simulink model "unlinear1130"  (R2021a)
settings: Solver=ode45  StartTime=0.0  StopTime=20  FixedStep=0  RelTol=1e-3  EnableMultiTasking=on
libraries: pid_lib x19, simulink x19
settings Model: NumberOfSteps=2  Creator=secn18  LastModifiedBy=HanDong
settings SolverCC: AlgebraicLoopSolver=TrustRegion
settings DataIOCC: LimitDataPoints=on  SaveFormat=Array  ReturnWorkspaceOutputs=off
settings OptimizationCC: LifeSpan=inf
settings DebuggingCC: SolverPrmCheckMsg=warning  SFUnexpectedBacktrackingDiag=warning  SFNoUnconditionalDefaultTransitionDiag=warning  SFExecutionAtInitializationDiag=none  SFMachineParentedDataDiag=warning  ArithmeticOperatorsInVariantConditions=warning
settings HardwareCC: ProdBitPerPointer=32  ProdBitPerSizeT=32  ProdBitPerPtrDiffT=32  ProdLargestAtomicFloat=None  ProdIntDivRoundTo=Undefined  ProdEndianess=Unspecified  ProdWordSize=32  ProdHWDeviceType=32-bit Generic
settings ModelReferenceCC: PropagateSignalLabelsOutOfModel=off
settings SFSimCC: SimUseLocalCustomCode=off  CustomCodeUndefinedFunction=UseInterfaceOnly
settings RTWCC: RTWUseLocalCustomCode=off
settings CodeAppCC: StateflowObjectComments=on
settings GRTTargetCC: TargetLangStandard=C89/C90 (ANSI)
settings ConfigComp: CovMetricSettings=dw  CovSaveCumulativeToWorkspaceVar=on  CovSaveSingleToWorkspaceVar=on  CovExternalEMLEnable=off  CovSFcnEnable=off

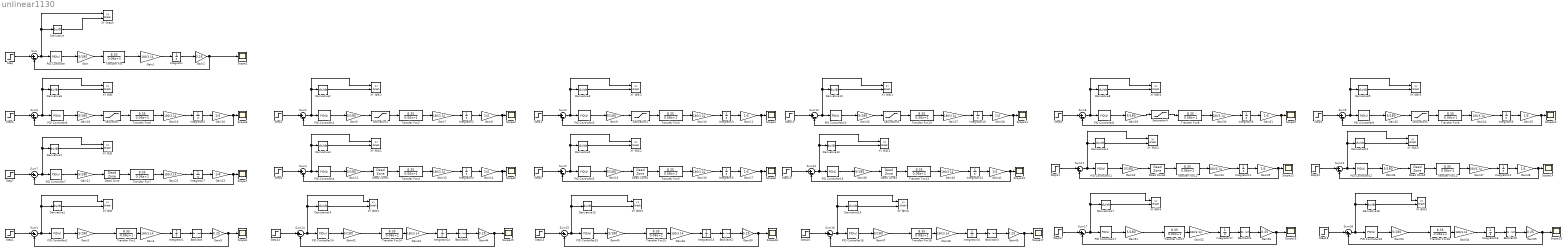
== system unlinear1130 ==
  Backlash : Backlash  BacklashWidth=0.2
  Backlash1 : Backlash  BacklashWidth=0.3
  Backlash2 : Backlash  BacklashWidth=0.4
  Backlash3 : Backlash  BacklashWidth=0.5
  Backlash4 : Backlash  BacklashWidth=1.2
  Backlash5 : Backlash  BacklashWidth=5
  Dead Zone : DeadZone  LowerValue=-0.2  UpperValue=0.2  SaturateOnIntegerOverflow=on
  Dead Zone1 : DeadZone  LowerValue=-0.3  UpperValue=0.3  SaturateOnIntegerOverflow=on
  Dead Zone2 : DeadZone  LowerValue=-0.4  UpperValue=0.4  SaturateOnIntegerOverflow=on
  Dead Zone3 : DeadZone  LowerValue=-1  UpperValue=1  SaturateOnIntegerOverflow=on
  Dead Zone4 : DeadZone  LowerValue=-5  UpperValue=5  SaturateOnIntegerOverflow=on
  Dead Zone5 : DeadZone  LowerValue=-10  UpperValue=10  SaturateOnIntegerOverflow=on
  Derivative{,1..18} (19 alike) : Derivative
  Gain{,3,6,9,12,15,18,21,26,29,32..33,36,39,42,45,47,51,53} (19 alike) : Gain  Gain=5/180
  Gain{1,4,7,10,13,16,19,22,24,27,30,34,37,40,43,46,48,52,54} (19 alike) : Gain  Gain=180/3.14
  Gain{8,11,14,17,20,23,25,28,31,35,38,41} (12 alike) : Gain  Gain=1/4
  Gain{2,5,44,49..50,55..56} (7 alike) : Gain  Gain=0.25
  Integrator{,1..18} (19 alike) : Integrator
  PID Controller : pid_lib/PID Controller  Controller=PID  Form=Parallel  TimeDomain=Continuous-time  UseExternalTs=off  SampleTime=1  IntegratorMethod=Forward Euler  FilterMethod=Forward Euler  ControllerParametersSource=internal  P=4  I=2  D=0.1  UseFilter=on  N=100  TunerSelectOption=Transfer Function Based (PID Tuner App)  InitialConditionSource=internal  InitialConditionForIntegrator=0  InitialConditionForFilter=0  DifferentiatorICPrevScaledInput=0  ExternalReset=none  TrackingMode=off  Kt=1  LimitOutput=off  SatLimitsSource=internal  UpperSaturationLimit=inf  LowerSaturationLimit=-inf  LinearizeAsGain=on  AntiWindupMode=none  Kb=1  POutMin=[]  POutMax=[]  IOutMin=[]  IOutMax=[]  DOutMin=[]  DOutMax=[]  NOutMin=[]  NOutMax=[]  SumOutMin=[]  SumOutMax=[]  SaturationOutMin=[]  SaturationOutMax=[]  PParamMin=[]  PParamMax=[]  IParamMin=[]  IParamMax=[]  DParamMin=[]  DParamMax=[]  NParamMin=[]  NParamMax=[]  KbParamMin=[]  KbParamMax=[]  KtParamMin=[]  KtParamMax=[]  KbOutMin=[]  KbOutMax=[]  KtOutMin=[]  KtOutMax=[]  IntegratorOutMin=[]  IntegratorOutMax=[]  FilterOutMin=[]  FilterOutMax=[]  SumI1OutMin=[]  SumI1OutMax=[]  SumI2OutMin=[]  SumI2OutMax=[]  SumI3OutMin=[]  SumI3OutMax=[]  SumI4OutMin=[]  SumI4OutMax=[]  SumDOutMin=[]  SumDOutMax=[]  DifferentiatorOutMin=[]  DifferentiatorOutMax=[]  FilterDiffOutCoefMin=[]  FilterDiffOutCoefMax=[]  ReciprocalOutMin=[]  ReciprocalOutMax=[]  SumDenOutMin=[]  SumDenOutMax=[]  SumNumOutMin=[]  SumNumOutMax=[]  DivideOutMin=[]  DivideOutMax=[]  UdiffTsProdOutMin=[]  UdiffTsProdOutMax=[]  NTsProdOutMin=[]  NTsProdOutMax=[]  UintegralTsProdOutMin=[]  UintegralTsProdOutMax=[]  UngainTsProdOutMin=[]  UngainTsProdOutMax=[]  IntegratorContinuousStateAttributes=''  IntegratorStateMustResolveToSignalObject=off  IntegratorRTWStateStorageClass=Auto  FilterContinuousStateAttributes=''  FilterStateMustResolveToSignalObject=off  FilterRTWStateStorageClass=Auto  ParallelPVariant=InternalParameters  IdealPVariant=Disabled  IVariant=InternalParameters  DVariant=InternalParameters  IntegratorVariant=Continuous  SatVariant=Disabled  AWVariant=Passthrough  PCopyVariant=Disabled  TRVariant=Disabled  FdbkBlocksVariant=Forward  IdealPFdbkVariant=Disabled  SatFdbkVariant=Disabled  DerivativeFilterVariant=ContFilter  NVariant=InternalParameters  NCopyVariant=Disabled  FilterICVariant=InternalICsFilter  IntegratorICVariant=InternalICs  ExternalResetVariant=Disabled  TRSumVariant=Passthrough  SumFdbkVariant=Disabled  SumVariant=Sum_PID  TsampFilterVariant=InternalTs  TsampNgainVariant=Passthrough  TsampIntegralVariant=Passthrough  ExternalSaturationOutDataTypeStr=Inherit: Same as second input
  PID Controller{1,14..18} (6 alike) : pid_lib/PID Controller  Controller=PID  Form=Parallel  TimeDomain=Continuous-time  UseExternalTs=off  SampleTime=1  IntegratorMethod=Forward Euler  FilterMethod=Forward Euler  ControllerParametersSource=internal  P=20  I=0  D=0.1  UseFilter=on  N=100  TunerSelectOption=Transfer Function Based (PID Tuner App)  InitialConditionSource=internal  InitialConditionForIntegrator=0  InitialConditionForFilter=0  DifferentiatorICPrevScaledInput=0  ExternalReset=none  TrackingMode=off  Kt=1  LimitOutput=off  SatLimitsSource=internal  UpperSaturationLimit=inf  LowerSaturationLimit=-inf  LinearizeAsGain=on  AntiWindupMode=none  Kb=1  POutMin=[]  POutMax=[]  IOutMin=[]  IOutMax=[]  DOutMin=[]  DOutMax=[]  NOutMin=[]  NOutMax=[]  SumOutMin=[]  SumOutMax=[]  SaturationOutMin=[]  SaturationOutMax=[]  PParamMin=[]  PParamMax=[]  IParamMin=[]  IParamMax=[]  DParamMin=[]  DParamMax=[]  NParamMin=[]  NParamMax=[]  KbParamMin=[]  KbParamMax=[]  KtParamMin=[]  KtParamMax=[]  KbOutMin=[]  KbOutMax=[]  KtOutMin=[]  KtOutMax=[]  IntegratorOutMin=[]  IntegratorOutMax=[]  FilterOutMin=[]  FilterOutMax=[]  SumI1OutMin=[]  SumI1OutMax=[]  SumI2OutMin=[]  SumI2OutMax=[]  SumI3OutMin=[]  SumI3OutMax=[]  SumI4OutMin=[]  SumI4OutMax=[]  SumDOutMin=[]  SumDOutMax=[]  DifferentiatorOutMin=[]  DifferentiatorOutMax=[]  FilterDiffOutCoefMin=[]  FilterDiffOutCoefMax=[]  ReciprocalOutMin=[]  ReciprocalOutMax=[]  SumDenOutMin=[]  SumDenOutMax=[]  SumNumOutMin=[]  SumNumOutMax=[]  DivideOutMin=[]  DivideOutMax=[]  UdiffTsProdOutMin=[]  UdiffTsProdOutMax=[]  NTsProdOutMin=[]  NTsProdOutMax=[]  UintegralTsProdOutMin=[]  UintegralTsProdOutMax=[]  UngainTsProdOutMin=[]  UngainTsProdOutMax=[]  IntegratorContinuousStateAttributes=''  IntegratorStateMustResolveToSignalObject=off  IntegratorRTWStateStorageClass=Auto  FilterContinuousStateAttributes=''  FilterStateMustResolveToSignalObject=off  FilterRTWStateStorageClass=Auto  ParallelPVariant=InternalParameters  IdealPVariant=Disabled  IVariant=InternalParameters  DVariant=InternalParameters  IntegratorVariant=Continuous  SatVariant=Disabled  AWVariant=Passthrough  PCopyVariant=Disabled  TRVariant=Disabled  FdbkBlocksVariant=Forward  IdealPFdbkVariant=Disabled  SatFdbkVariant=Disabled  DerivativeFilterVariant=ContFilter  NVariant=InternalParameters  NCopyVariant=Disabled  FilterICVariant=InternalICsFilter  IntegratorICVariant=InternalICs  ExternalResetVariant=Disabled  TRSumVariant=Passthrough  SumFdbkVariant=Disabled  SumVariant=Sum_PID  TsampFilterVariant=InternalTs  TsampNgainVariant=Passthrough  TsampIntegralVariant=Passthrough  ExternalSaturationOutDataTypeStr=Inherit: Same as second input
  PID Controller{2..3,6,8..10} (6 alike) : pid_lib/PID Controller  Controller=PID  Form=Parallel  TimeDomain=Continuous-time  UseExternalTs=off  SampleTime=-1  IntegratorMethod=Forward Euler  FilterMethod=Forward Euler  ControllerParametersSource=internal  P=2  I=15  D=0.1  UseFilter=on  N=100  TunerSelectOption=Transfer Function Based (PID Tuner App)  InitialConditionSource=internal  InitialConditionForIntegrator=0  InitialConditionForFilter=0  DifferentiatorICPrevScaledInput=0  ExternalReset=none  TrackingMode=off  Kt=1  LimitOutput=off  SatLimitsSource=internal  UpperSaturationLimit=inf  LowerSaturationLimit=-inf  LinearizeAsGain=on  AntiWindupMode=none  Kb=1  POutMin=[]  POutMax=[]  IOutMin=[]  IOutMax=[]  DOutMin=[]  DOutMax=[]  NOutMin=[]  NOutMax=[]  SumOutMin=[]  SumOutMax=[]  SaturationOutMin=[]  SaturationOutMax=[]  PParamMin=[]  PParamMax=[]  IParamMin=[]  IParamMax=[]  DParamMin=[]  DParamMax=[]  NParamMin=[]  NParamMax=[]  KbParamMin=[]  KbParamMax=[]  KtParamMin=[]  KtParamMax=[]  KbOutMin=[]  KbOutMax=[]  KtOutMin=[]  KtOutMax=[]  IntegratorOutMin=[]  IntegratorOutMax=[]  FilterOutMin=[]  FilterOutMax=[]  SumI1OutMin=[]  SumI1OutMax=[]  SumI2OutMin=[]  SumI2OutMax=[]  SumI3OutMin=[]  SumI3OutMax=[]  SumI4OutMin=[]  SumI4OutMax=[]  SumDOutMin=[]  SumDOutMax=[]  DifferentiatorOutMin=[]  DifferentiatorOutMax=[]  FilterDiffOutCoefMin=[]  FilterDiffOutCoefMax=[]  ReciprocalOutMin=[]  ReciprocalOutMax=[]  SumDenOutMin=[]  SumDenOutMax=[]  SumNumOutMin=[]  SumNumOutMax=[]  DivideOutMin=[]  DivideOutMax=[]  UdiffTsProdOutMin=[]  UdiffTsProdOutMax=[]  NTsProdOutMin=[]  NTsProdOutMax=[]  UintegralTsProdOutMin=[]  UintegralTsProdOutMax=[]  UngainTsProdOutMin=[]  UngainTsProdOutMax=[]  IntegratorContinuousStateAttributes=''  IntegratorStateMustResolveToSignalObject=off  IntegratorRTWStateStorageClass=Auto  FilterContinuousStateAttributes=''  FilterStateMustResolveToSignalObject=off  FilterRTWStateStorageClass=Auto  ParallelPVariant=InternalParameters  IdealPVariant=Disabled  IVariant=InternalParameters  DVariant=InternalParameters  IntegratorVariant=Continuous  SatVariant=Disabled  AWVariant=Passthrough  PCopyVariant=Disabled  TRVariant=Disabled  FdbkBlocksVariant=Forward  IdealPFdbkVariant=Disabled  SatFdbkVariant=Disabled  DerivativeFilterVariant=ContFilter  NVariant=InternalParameters  NCopyVariant=Disabled  FilterICVariant=InternalICsFilter  IntegratorICVariant=InternalICs  ExternalResetVariant=Disabled  TRSumVariant=Passthrough  SumFdbkVariant=Disabled  SumVariant=Sum_PID  TsampFilterVariant=InternalTs  TsampNgainVariant=Passthrough  TsampIntegralVariant=Passthrough  ExternalSaturationOutDataTypeStr=Inherit: Same as second input
  PID Controller{4..5,7,11..13} (6 alike) : pid_lib/PID Controller  Controller=PID  Form=Parallel  TimeDomain=Continuous-time  UseExternalTs=off  SampleTime=-1  IntegratorMethod=Forward Euler  FilterMethod=Forward Euler  ControllerParametersSource=internal  P=2  I=15  D=0  UseFilter=on  N=100  TunerSelectOption=Transfer Function Based (PID Tuner App)  InitialConditionSource=internal  InitialConditionForIntegrator=0  InitialConditionForFilter=0  DifferentiatorICPrevScaledInput=0  ExternalReset=none  TrackingMode=off  Kt=1  LimitOutput=off  SatLimitsSource=internal  UpperSaturationLimit=inf  LowerSaturationLimit=-inf  LinearizeAsGain=on  AntiWindupMode=none  Kb=1  POutMin=[]  POutMax=[]  IOutMin=[]  IOutMax=[]  DOutMin=[]  DOutMax=[]  NOutMin=[]  NOutMax=[]  SumOutMin=[]  SumOutMax=[]  SaturationOutMin=[]  SaturationOutMax=[]  PParamMin=[]  PParamMax=[]  IParamMin=[]  IParamMax=[]  DParamMin=[]  DParamMax=[]  NParamMin=[]  NParamMax=[]  KbParamMin=[]  KbParamMax=[]  KtParamMin=[]  KtParamMax=[]  KbOutMin=[]  KbOutMax=[]  KtOutMin=[]  KtOutMax=[]  IntegratorOutMin=[]  IntegratorOutMax=[]  FilterOutMin=[]  FilterOutMax=[]  SumI1OutMin=[]  SumI1OutMax=[]  SumI2OutMin=[]  SumI2OutMax=[]  SumI3OutMin=[]  SumI3OutMax=[]  SumI4OutMin=[]  SumI4OutMax=[]  SumDOutMin=[]  SumDOutMax=[]  DifferentiatorOutMin=[]  DifferentiatorOutMax=[]  FilterDiffOutCoefMin=[]  FilterDiffOutCoefMax=[]  ReciprocalOutMin=[]  ReciprocalOutMax=[]  SumDenOutMin=[]  SumDenOutMax=[]  SumNumOutMin=[]  SumNumOutMax=[]  DivideOutMin=[]  DivideOutMax=[]  UdiffTsProdOutMin=[]  UdiffTsProdOutMax=[]  NTsProdOutMin=[]  NTsProdOutMax=[]  UintegralTsProdOutMin=[]  UintegralTsProdOutMax=[]  UngainTsProdOutMin=[]  UngainTsProdOutMax=[]  IntegratorContinuousStateAttributes=''  IntegratorStateMustResolveToSignalObject=off  IntegratorRTWStateStorageClass=Auto  FilterContinuousStateAttributes=''  FilterStateMustResolveToSignalObject=off  FilterRTWStateStorageClass=Auto  ParallelPVariant=InternalParameters  IdealPVariant=Disabled  IVariant=InternalParameters  DVariant=InternalParameters  IntegratorVariant=Continuous  SatVariant=Disabled  AWVariant=Passthrough  PCopyVariant=Disabled  TRVariant=Disabled  FdbkBlocksVariant=Forward  IdealPFdbkVariant=Disabled  SatFdbkVariant=Disabled  DerivativeFilterVariant=ContFilter  NVariant=InternalParameters  NCopyVariant=Disabled  FilterICVariant=InternalICsFilter  IntegratorICVariant=InternalICs  ExternalResetVariant=Disabled  TRSumVariant=Passthrough  SumFdbkVariant=Disabled  SumVariant=Sum_PID  TsampFilterVariant=InternalTs  TsampNgainVariant=Passthrough  TsampIntegralVariant=Passthrough  ExternalSaturationOutDataTypeStr=Inherit: Same as second input
  Saturation : Saturate  UpperLimit=0.1  LowerLimit=-0.1
  Saturation1 : Saturate  UpperLimit=0.3  LowerLimit=-0.3
  Saturation2 : Saturate  UpperLimit=0.4  LowerLimit=-0.4
  Saturation3 : Saturate
  Saturation4 : Saturate  UpperLimit=0.6  LowerLimit=-0.6
  Saturation5 : Saturate  UpperLimit=0.7  LowerLimit=-0.7
  Scope{1..19} (19 alike) : Scope
  Step{,1..18} (19 alike) : Step  Time=0  SampleTime=0
  Sum{,1..18} (19 alike) : Sum  Inputs=|+-
  Transfer Fcn{,1..18} (19 alike) : TransferFcn  Numerator=[8.35]  Denominator=[0.06 1]
  XY Graph : simulink/Sinks/XY Graph  xmin=-1.5  xmax=1.5  ymin=-40  ymax=40  st=0
  XY 死区{,1..5} (6 alike) : simulink/Sinks/XY Graph  xmin=-1.5  xmax=1.5  ymin=-7  ymax=7  st=0
  XY 滞环{,1..5} (6 alike) : simulink/Sinks/XY Graph  xmin=-1.5  xmax=1.5  ymin=-40  ymax=40  st=0
  XY 饱和{,1..4} (5 alike) : simulink/Sinks/XY Graph  xmin=-1.5  xmax=1.5  ymin=-20  ymax=7  st=0
  XY 饱和5 : simulink/Sinks/XY Graph  xmin=-5  xmax=5  ymin=-20  ymax=7  st=0
  wires:
  Step/1 -> Sum/1
  Sum/1 -> XY Graph/1, Derivative/1, PID Controller/1
  PID Controller/1 -> Gain/1
  Gain/1 -> Transfer Fcn/1
  Transfer Fcn/1 -> Gain1/1
  Gain1/1 -> Integrator/1
  Integrator/1 -> Gain2/1
  Gain2/1 -> Scope2/1, Sum/2
  Derivative/1 -> XY Graph/2
  Step1/1 -> Sum1/1
  Sum1/1 -> XY 滞环/1, Derivative1/1, PID Controller1/1
  PID Controller1/1 -> Gain3/1
  Transfer Fcn1/1 -> Gain4/1
  Gain4/1 -> Integrator1/1
  Integrator1/1 -> Backlash/1
  Gain5/1 -> Scope1/1, Sum1/2
  Derivative1/1 -> XY 滞环/2
  Gain3/1 -> Transfer Fcn1/1
  Backlash/1 -> Gain5/1
  Step6/1 -> Sum6/1
  Sum6/1 -> XY 饱和/1, Derivative6/1, PID Controller6/1
  PID Controller6/1 -> Gain18/1
  Gain18/1 -> Saturation/1
  Saturation/1 -> Transfer Fcn6/1
  Transfer Fcn6/1 -> Gain19/1
  Gain19/1 -> Integrator6/1
  Integrator6/1 -> Gain20/1
  Gain20/1 -> Sum6/2, Scope6/1
  Derivative6/1 -> XY 饱和/2
  Step7/1 -> Sum7/1
  Derivative7/1 -> XY 死区/2
  Gain23/1 -> Sum7/2, Scope7/1
  Transfer Fcn7/1 -> Gain22/1
  Gain21/1 -> Dead Zone/1
  Integrator7/1 -> Gain23/1
  Sum7/1 -> XY 死区/1, Derivative7/1, PID Controller7/1
  PID Controller7/1 -> Gain21/1
  Dead Zone/1 -> Transfer Fcn7/1
  Gain22/1 -> Integrator7/1
  Step2/1 -> Sum2/1
  Derivative2/1 -> XY 饱和2/2
  Gain8/1 -> Sum2/2, Scope3/1
  Transfer Fcn2/1 -> Gain7/1
  Gain6/1 -> Saturation1/1
  Integrator2/1 -> Gain8/1
  Sum2/1 -> XY 饱和2/1, Derivative2/1, PID Controller2/1
  PID Controller2/1 -> Gain6/1
  Saturation1/1 -> Transfer Fcn2/1
  Gain7/1 -> Integrator2/1
  Gain10/1 -> Integrator3/1
  PID Controller3/1 -> Gain9/1
  Sum3/1 -> XY 饱和3/1, Derivative3/1, PID Controller3/1
  Gain9/1 -> Saturation2/1
  Integrator3/1 -> Gain11/1
  Transfer Fcn3/1 -> Gain10/1
  Gain11/1 -> Sum3/2, Scope4/1
  Derivative3/1 -> XY 饱和3/2
  Saturation2/1 -> Transfer Fcn3/1
  Step3/1 -> Sum3/1
  Gain12/1 -> Dead Zone1/1
  Dead Zone1/1 -> Transfer Fcn4/1
  Sum4/1 -> XY 死区1/1, Derivative4/1, PID Controller4/1
  Gain13/1 -> Integrator4/1
  Transfer Fcn4/1 -> Gain13/1
  Derivative4/1 -> XY 死区1/2
  Integrator4/1 -> Gain14/1
  Step4/1 -> Sum4/1
  PID Controller4/1 -> Gain12/1
  Gain14/1 -> Sum4/2, Scope5/1
  Gain15/1 -> Dead Zone2/1
  Dead Zone2/1 -> Transfer Fcn5/1
  Sum5/1 -> XY 死区2/1, Derivative5/1, PID Controller5/1
  Gain16/1 -> Integrator5/1
  Transfer Fcn5/1 -> Gain16/1
  Derivative5/1 -> XY 死区2/2
  Integrator5/1 -> Gain17/1
  Step5/1 -> Sum5/1
  PID Controller5/1 -> Gain15/1
  Gain17/1 -> Sum5/2, Scope8/1
  Gain30/1 -> Integrator8/1
  Sum8/1 -> XY 饱和4/1, Derivative8/1, PID Controller8/1
  Gain29/1 -> Saturation4/1
  Gain31/1 -> Sum8/2, Scope9/1
  Derivative8/1 -> XY 饱和4/2
  Saturation4/1 -> Transfer Fcn8/1
  Step8/1 -> Sum8/1
  Step9/1 -> Sum9/1
  Transfer Fcn9/1 -> Gain24/1
  Sum9/1 -> XY 饱和5/1, Derivative9/1, PID Controller9/1
  Gain25/1 -> Sum9/2, Scope10/1
  Derivative9/1 -> XY 饱和5/2
  Saturation5/1 -> Transfer Fcn9/1
  Gain32/1 -> Saturation5/1
  Integrator8/1 -> Gain31/1
  PID Controller9/1 -> Gain32/1
  Gain24/1 -> Integrator9/1
  PID Controller8/1 -> Gain29/1
  Step10/1 -> Sum10/1
  Derivative10/1 -> XY 饱和1/2
  Gain28/1 -> Sum10/2, Scope11/1
  Integrator9/1 -> Gain25/1
  Transfer Fcn8/1 -> Gain30/1
  Transfer Fcn10/1 -> Gain27/1
  Gain26/1 -> Saturation3/1
  Integrator10/1 -> Gain28/1
  Sum10/1 -> XY 饱和1/1, Derivative10/1, PID Controller10/1
  PID Controller10/1 -> Gain26/1
  Saturation3/1 -> Transfer Fcn10/1
  Gain27/1 -> Integrator10/1
  Dead Zone5/1 -> Transfer Fcn12/1
  Derivative11/1 -> XY 死区4/2
  PID Controller11/1 -> Gain33/1
  Transfer Fcn11/1 -> Gain34/1
  Gain35/1 -> Sum11/2, Scope12/1
  Dead Zone4/1 -> Transfer Fcn11/1
  Gain33/1 -> Dead Zone4/1
  Gain39/1 -> Dead Zone3/1
  Sum11/1 -> XY 死区4/1, Derivative11/1, PID Controller11/1
  Dead Zone3/1 -> Transfer Fcn13/1
  Sum13/1 -> XY 死区3/1, Derivative13/1, PID Controller13/1
  Gain40/1 -> Integrator13/1
  Gain41/1 -> Sum13/2, Scope13/1
  Gain36/1 -> Dead Zone5/1
  Derivative13/1 -> XY 死区3/2
  PID Controller13/1 -> Gain39/1
  Integrator13/1 -> Gain41/1
  Step13/1 -> Sum13/1
  Integrator11/1 -> Gain35/1
  Gain38/1 -> Sum12/2, Scope14/1
  Step12/1 -> Sum12/1
  Gain37/1 -> Integrator12/1
  Gain34/1 -> Integrator11/1
  Integrator12/1 -> Gain38/1
  Derivative12/1 -> XY 死区5/2
  Sum12/1 -> XY 死区5/1, Derivative12/1, PID Controller12/1
  PID Controller12/1 -> Gain36/1
  Transfer Fcn12/1 -> Gain37/1
  Transfer Fcn13/1 -> Gain40/1
  Step11/1 -> Sum11/1
  Step14/1 -> Sum14/1
  Gain43/1 -> Integrator14/1
  Integrator14/1 -> Backlash1/1
  PID Controller14/1 -> Gain42/1
  Backlash1/1 -> Gain44/1
  Derivative14/1 -> XY 滞环1/2
  Transfer Fcn14/1 -> Gain43/1
  Gain44/1 -> Scope15/1, Sum14/2
  Gain42/1 -> Transfer Fcn14/1
  Sum14/1 -> XY 滞环1/1, Derivative14/1, PID Controller14/1
  Integrator16/1 -> Backlash3/1
  Derivative16/1 -> XY 滞环3/2
  Transfer Fcn16/1 -> Gain48/1
  Step16/1 -> Sum16/1
  Step15/1 -> Sum15/1
  Gain46/1 -> Integrator15/1
  Integrator15/1 -> Backlash2/1
  PID Controller15/1 -> Gain45/1
  PID Controller16/1 -> Gain47/1
  Backlash3/1 -> Gain49/1
  Backlash2/1 -> Gain50/1
  Derivative15/1 -> XY 滞环2/2
  Sum16/1 -> XY 滞环3/1, Derivative16/1, PID Controller16/1
  Transfer Fcn15/1 -> Gain46/1
  Gain48/1 -> Integrator16/1
  Gain47/1 -> Transfer Fcn16/1
  Gain49/1 -> Scope17/1, Sum16/2
  Gain50/1 -> Scope16/1, Sum15/2
  Gain45/1 -> Transfer Fcn15/1
  Sum15/1 -> XY 滞环2/1, Derivative15/1, PID Controller15/1
  Integrator18/1 -> Backlash5/1
  Derivative18/1 -> XY 滞环5/2
  Transfer Fcn18/1 -> Gain54/1
  Step18/1 -> Sum18/1
  Step17/1 -> Sum17/1
  Gain52/1 -> Integrator17/1
  Integrator17/1 -> Backlash4/1
  PID Controller17/1 -> Gain51/1
  PID Controller18/1 -> Gain53/1
  Backlash5/1 -> Gain55/1
  Backlash4/1 -> Gain56/1
  Derivative17/1 -> XY 滞环4/2
  Sum18/1 -> XY 滞环5/1, Derivative18/1, PID Controller18/1
  Transfer Fcn17/1 -> Gain52/1
  Gain54/1 -> Integrator18/1
  Gain53/1 -> Transfer Fcn18/1
  Gain55/1 -> Scope19/1, Sum18/2
  Gain56/1 -> Scope18/1, Sum17/2
  Gain51/1 -> Transfer Fcn17/1
  Sum17/1 -> XY 滞环4/1, Derivative17/1, PID Controller17/1
